simulink model "Tv_VSI"  (Simulink 8.1)
settings: Solver=ode23t  StartTime=0.0  StopTime=0.5  MaxStep=25e-6  RelTol=1e-4  AbsTol=1e-5
values from neighbouring files (symbols this model uses):
  C = 1*31.5e-6    (= 3.15e-05)    [TVSI_vil_tf_cal_sim_comp_frd_model.m]    (also in VSI_ol_init.m = 3.13e-05; VSI_ol_tf_cal_sim_comp_frd_model.m = 3.13e-05; Zac_VSI.m = 3.18e-05; Zdc_VSI.m)
  CR = .2    (= 0.2)    [TVSI_vil_tf_cal_sim_comp_frd_model.m]    (also in Zac_VSI.m = 1)
  Gdel = Gsvm    [TVSI_vil_tf_cal_sim_comp_frd_model.m]    (also in VSI_ol_init.m; VSI_ol_tf_cal_sim_comp_frd_model.m; Zac_VSI.m; Zdc_VSI.m)
  Ki = tf_filter_dq    [TVSI_vil_tf_cal_sim_comp_frd_model.m]    (also in VSI_ol_init.m; Zac_VSI.m; Zdc_VSI.m)
  kii = Kii_VSI/270    (= 0)    [TVSI_vil_tf_cal_sim_comp_frd_model.m]    (also in Zac_VSI.m; Zdc_VSI.m = 121.0095)
  kiv = Kiv_VSI    (= 523.598775598)    [TVSI_vil_tf_cal_sim_comp_frd_model.m]    (also in Zac_VSI.m = 78.5398163397; Zdc_VSI.m = 130.8997)
  kpi = Kpi_VSI/270    (= 0.0116355283466)    [TVSI_vil_tf_cal_sim_comp_frd_model.m]    (also in Zac_VSI.m = 0.00407243492132; Zdc_VSI.m = 0.0465)
  kpv = Kpv_VSI    (= 0.197920337176)    [TVSI_vil_tf_cal_sim_comp_frd_model.m]    (also in Zac_VSI.m = 0.0290283161192; Zdc_VSI.m = 0.0495)
  Kv = tf_filter_dq    [TVSI_vil_tf_cal_sim_comp_frd_model.m]    (also in VSI_ol_init.m; Zac_VSI.m; Zdc_VSI.m)
  L = 1.0e-3    (= 0.001)    [TVSI_vil_tf_cal_sim_comp_frd_model.m]    (also in VSI_ol_init.m; VSI_ol_tf_cal_sim_comp_frd_model.m; Zac_VSI.m = 0.000506643235509; Zdc_VSI.m)
  R = 12    [TVSI_vil_tf_cal_sim_comp_frd_model.m]    (also in VSI_ol_init.m = 15; VSI_ol_tf_cal_sim_comp_frd_model.m = 12000; Zac_VSI.m; Zdc_VSI.m)
  RL = 0.13    [TVSI_vil_tf_cal_sim_comp_frd_model.m]    (also in VSI_ol_init.m = 0.15; VSI_ol_tf_cal_sim_comp_frd_model.m = 0.15; Zac_VSI.m = 0.06; Zdc_VSI.m)
  Vdc = 270    [TVSI_vil_tf_cal_sim_comp_frd_model.m]    (also in VSI_ol_init.m; VSI_ol_tf_cal_sim_comp_frd_model.m; Zac_VSI.m; Zdc_VSI.m)
  Vdref = Vsdq(1)    [TVSI_vil_tf_cal_sim_comp_frd_model.m]    (also in VSI_ol_init.m; VSI_ol_tf_cal_sim_comp_frd_model.m; Zac_VSI.m; Zdc_VSI.m)
  Vqref = Vsdq(2)    [TVSI_vil_tf_cal_sim_comp_frd_model.m]    (also in VSI_ol_init.m; VSI_ol_tf_cal_sim_comp_frd_model.m; Zac_VSI.m; Zdc_VSI.m)
  w = 500*2*pi    (= 3141.59265359)    [JF_CMOD.m]    (also in JF_SMOD.m; TVSI_vil_tf_cal_sim_comp_frd_model.m = 376.991118431; VSI_ol_init.m = 2513.27412287; VSI_ol_tf_cal_sim_comp_frd_model.m = 376.991118431)
libraries: powerlib x28, cstblocks x12
settings Model: Creator=marko  LastModifiedBy=wenbo  BufferReuse=off
settings OptimizationCC: BlockReduction=off  InlineParams=on  BufferReuse=off
settings DebuggingCC: AlgebraicLoopMsg=none  SolverPrmCheckMsg=none  UnconnectedInputMsg=none  UnconnectedOutputMsg=none  UnconnectedLineMsg=none

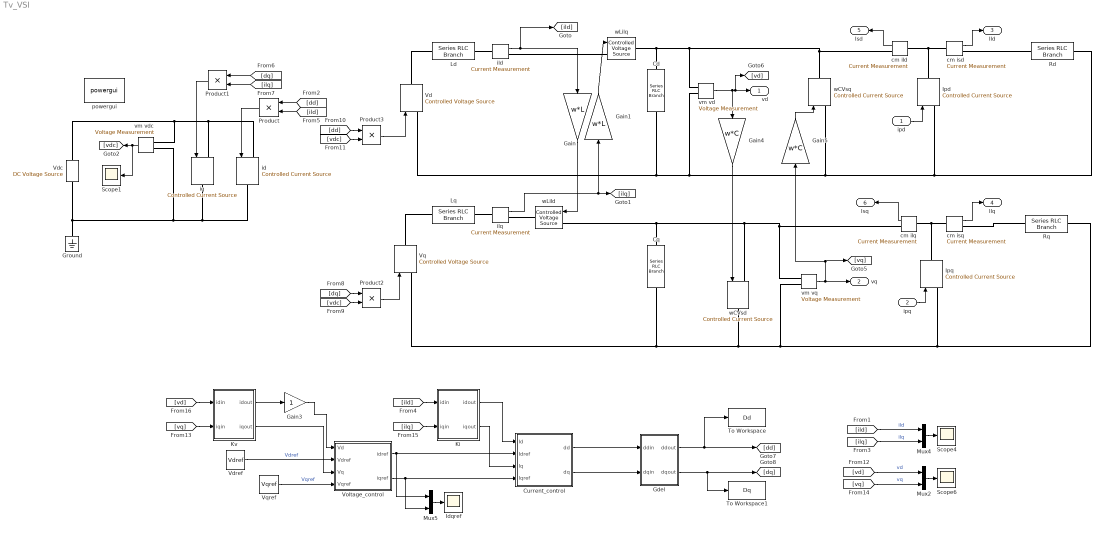
== system Tv_VSI ==
  ipd : Inport
  ipq : Inport  Port=2
  Cd : powerlib/Elements/Series RLC Branch  LConnTagsString=__new0  RConnTagsString=__new0  BranchType=RC  Resistance=CR  Inductance=1e-3  SetiL0=off  InitialCurrent=0  Capacitance=C  Setx0=off  InitialVoltage=0  Measurements=None
  Cq : powerlib/Elements/Series RLC Branch  LConnTagsString=__new0  RConnTagsString=__new0  BranchType=RC  Resistance=CR  Inductance=1e-3  SetiL0=off  InitialCurrent=0  Capacitance=C  Setx0=off  InitialVoltage=0  Measurements=None
  Current_control : Subsystem
  Gain : Gain  Gain=w*L
  Gain1 : Gain  Gain=w*L
  Gain3 : Gain
  Gain4 : Gain  Gain=w*C
  Gain5 : Gain  Gain=w*C
  Gdel : Subsystem
  Ground : powerlib/Elements/Ground  LConnTagsString=a
  Idqref : Scope
      settings: YMin=4.4  YMax=5.35  SaveName=ildq_matlab8
  Ipd : powerlib/Electrical Sources/Controlled Current Source  Initialize=on  Source_Type=AC  Amplitude=0  Phase=0  Frequency=0  Measurements=None
  Ipq : powerlib/Electrical Sources/Controlled Current Source  Initialize=on  Source_Type=AC  Amplitude=0  Phase=0  Frequency=0  Measurements=None
  Ki : Subsystem
  Kv : Subsystem
  Ld : powerlib/Elements/Series RLC Branch  LConnTagsString=__new0  RConnTagsString=__new0  BranchType=RL  Resistance=RL  Inductance=L  SetiL0=off  InitialCurrent=0  Capacitance=1e-6  Setx0=off  InitialVoltage=0  Measurements=None
  Lq : powerlib/Elements/Series RLC Branch  LConnTagsString=__new0  RConnTagsString=__new0  BranchType=RL  Resistance=RL  Inductance=L  SetiL0=off  InitialCurrent=0  Capacitance=1e-6  Setx0=off  InitialVoltage=0  Measurements=None
  Mux2 : Mux  Inputs=2
  Mux4 : Mux  Inputs=2
  Mux5 : Mux  Inputs=2
  Product{,1..3} (4 alike) : Product  RndMeth=Zero
  Rd : powerlib/Elements/Series RLC Branch  LConnTagsString=__new0  RConnTagsString=__new0  BranchType=R  Resistance=R  Inductance=1e-3  SetiL0=off  InitialCurrent=0  Capacitance=1e-6  Setx0=off  InitialVoltage=0  Measurements=None
  Rq : powerlib/Elements/Series RLC Branch  LConnTagsString=__new0  RConnTagsString=__new0  BranchType=R  Resistance=R  Inductance=1e-3  SetiL0=off  InitialCurrent=0  Capacitance=1e-6  Setx0=off  InitialVoltage=0  Measurements=None
  Scope1 : Scope
      settings: YMin=270  YMax=270  SaveName=ildq_matlab
  Scope4 : Scope
      settings: YMin=-0.25  YMax=5.25  SaveName=ildq_matlab3
  Scope6 : Scope
      settings: YMin=-10  YMax=130  SaveName=ildq_matlab4
  To Workspace : ToWorkspace  VariableName=Dd  SampleTime=-1
  To Workspace1 : ToWorkspace  VariableName=Dq  SampleTime=-1
  Vd : powerlib/Electrical Sources/Controlled Voltage Source  Initialize=on  Source_Type=DC  Amplitude=0  Phase=0  Frequency=0  Measurements=None
  Vdc : powerlib/Electrical Sources/DC Voltage Source  Amplitude=Vdc  Measurements=None
  Vdref : Constant  Value=Vdref
  Voltage_control : Subsystem
  Vq : powerlib/Electrical Sources/Controlled Voltage Source  Initialize=on  Source_Type=DC  Amplitude=0  Phase=0  Frequency=0  Measurements=None
  Vqref : Constant  Value=Vqref
  cm ild : powerlib/Measurements/Current Measurement  PhasorSimulation=off  OutputType=Complex  PSBequivalent=0
  cm ilq : powerlib/Measurements/Current Measurement  PhasorSimulation=off  OutputType=Complex  PSBequivalent=0
  cm isd : powerlib/Measurements/Current Measurement  PhasorSimulation=off  OutputType=Complex  PSBequivalent=0
  cm isq : powerlib/Measurements/Current Measurement  PhasorSimulation=off  OutputType=Complex  PSBequivalent=0
  id : powerlib/Electrical Sources/Controlled Current Source  Initialize=on  Source_Type=DC  Amplitude=0  Phase=0  Frequency=0  Measurements=None
  ild : powerlib/Measurements/Current Measurement  PhasorSimulation=off  OutputType=Complex  PSBequivalent=0
  ilq : powerlib/Measurements/Current Measurement  PhasorSimulation=off  OutputType=Complex  PSBequivalent=0
  iq : powerlib/Electrical Sources/Controlled Current Source  Initialize=on  Source_Type=DC  Amplitude=0  Phase=0  Frequency=0  Measurements=None
  powergui : powerlib/powergui  Priority=1  SimulationMode=Continuous  SolverType=Tustin  SampleTime=50e-6  frequency=60  SPID=off  DisableSnubberDevices=off  DisableRonSwitches=off  DisableVfSwitches=off  SwTol=0  Interpol=off  DisplayEquations=off  frequencyindice=0  Pbase=100e6  ErrMax=1e-4  Iterations=50  UnitsV=kV  UnitsW=MW  FunctionMessages=off  echomessages=off  HookPort=off  EnableUseOfTLC=off  x0status=blocks  RestoreLinks=warning  ResistiveCurrentMeasurement=off  Frange=[0:2:500]  Ylog=off  Xlog=on  ShowGrid=off  save=off  variable=ZData  ZoomFFT=on  StartTime=0.0  cycles=1  DisplayStyle=1  fundamental=60  FreqAxis=off  MaxFrequency=1000  frequencyindicesteady=1  RmsSteady=1  display=off  Ts=0  methode=off
  vm vd : powerlib/Measurements/Voltage Measurement  PhasorSimulation=off  OutputType=Complex  PSBequivalent=0
  vm vdc : powerlib/Measurements/Voltage Measurement  PhasorSimulation=off  OutputType=Complex  PSBequivalent=0
  vm vq : powerlib/Measurements/Voltage Measurement  PhasorSimulation=off  OutputType=Complex  PSBequivalent=0
  wCVsd : powerlib/Electrical Sources/Controlled Current Source  Initialize=on  Source_Type=DC  Amplitude=0  Phase=0  Frequency=0  Measurements=None
  wCVsq : powerlib/Electrical Sources/Controlled Current Source  Initialize=on  Source_Type=DC  Amplitude=0  Phase=0  Frequency=0  Measurements=None
  wLild : powerlib/Electrical Sources/Controlled Voltage Source  Initialize=on  Source_Type=DC  Amplitude=0  Phase=0  Frequency=0  Measurements=None
  wLilq : powerlib/Electrical Sources/Controlled Voltage Source  Initialize=on  Source_Type=DC  Amplitude=0  Phase=0  Frequency=0  Measurements=None
  vd : Outport
  vq : Outport  Port=2
  Ild : Outport  Port=3
  Ilq : Outport  Port=4
  Isd : Outport  Port=5
  Isq : Outport  Port=6
  wires:
  [ild] -> Mux4/1  "ild"
  [ilq] -> Mux4/2  "ilq"
  Mux4/1 -> Scope4/1
  [vd] -> Mux2/1  "vd"
  [vq] -> Mux2/2  "vq"
  Mux2/1 -> Scope6/1
  Voltage_control/2(iqref) -> Mux5/2, Current_control/4(Iqref)
  Gdel/1(ddout) -> [dd], To Workspace/1
  Gdel/2(dqout) -> [dq], To Workspace1/1
  Vqref/1 -> Voltage_control/4(Vqref)  "Vqref"
  Vdref/1 -> Voltage_control/2(Vdref)  "Vdref"
  Voltage_control/1(idref) -> Mux5/1, Current_control/2(Idref)
  Mux5/1 -> Idqref/1
  [ild] -> Ki/1(idin)
  [ilq] -> Ki/2(iqin)
  Ki/1(idout) -> Current_control/1(Id)
  Ki/2(iqout) -> Current_control/3(Iq)
  Current_control/1(dd) -> Gdel/1(ddin)
  Current_control/2(dq) -> Gdel/2(dqin)
  [vd] -> Kv/1(idin)
  [vq] -> Kv/2(iqin)
  Kv/2(iqout) -> Voltage_control/3(Vq)
  Kv/1(idout) -> Gain3/1
  Gain3/1 -> Voltage_control/1(Vd)
  Product1/1 -> iq/1
  [dq] -> Product2/1
  [vdc] -> Product2/2
  Product2/1 -> Vq/1
  [dd] -> Product3/1
  [vdc] -> Product3/2
  Product3/1 -> Vd/1
  vm vd/1 -> vd/1, [vd], Gain4/1
  vm vq/1 -> vq/1, Gain5/1, [vq]
  vm vdc/1 -> [vdc], Scope1/1
  ilq/1 -> [ilq], Gain1/1
  ild/1 -> Gain/1, [ild]
  Gain5/1 -> wCVsq/1
  [dd] -> Product/1
  [ild] -> Product/2
  [dq] -> Product1/1
  [ilq] -> Product1/2
  Product/1 -> id/1
  Gain/1 -> wLild/1
  Gain1/1 -> wLilq/1
  Gain4/1 -> wCVsd/1
  ipd/1 -> Ipd/1
  cm ild/1 -> Isd/1
  cm isd/1 -> Ild/1
  ipq/1 -> Ipq/1
  cm ilq/1 -> Isq/1
  cm isq/1 -> Ilq/1
  connections:
  vm vq/LConn2 -- Rq/RConn1 -- Ipq/LConn1 -- wCVsd/RConn1 -- Vq/LConn1 -- Cq/RConn1
  vm vdc/LConn2 -- Ground/LConn1 -- Vdc/LConn1 -- iq/RConn1 -- id/RConn1
  vm vq/LConn1 -- cm ilq/RConn1 -- wCVsd/LConn1 -- wLild/LConn1 -- Cq/LConn1
  vm vdc/LConn1 -- Vdc/RConn1 -- id/LConn1 -- iq/LConn1
  vm vd/LConn1 -- cm ild/RConn1 -- wCVsq/RConn1 -- Cd/LConn1 -- wLilq/RConn1
  vm vd/LConn2 -- Ipd/LConn1 -- Rd/RConn1 -- wCVsq/LConn1 -- Vd/LConn1 -- Cd/RConn1
  cm ild/LConn1 -- Ipd/RConn1 -- cm isd/LConn1
  cm ilq/LConn1 -- Ipq/RConn1 -- cm isq/LConn1
  wLild/RConn1 -- ilq/RConn1
  Ld/LConn1 -- Vd/RConn1
  ilq/LConn1 -- Lq/LConn1
  cm isd/RConn1 -- Rd/LConn1
  Lq/RConn1 -- Vq/RConn1
  wLilq/LConn1 -- ild/RConn1
  cm isq/RConn1 -- Rq/LConn1
  ild/LConn1 -- Ld/RConn1

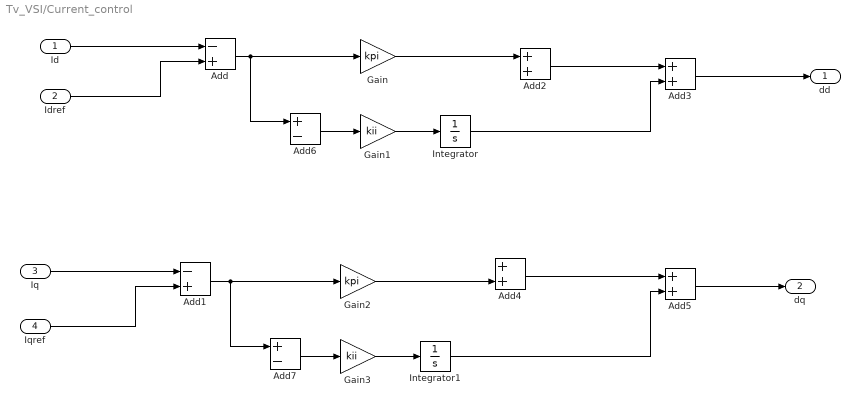
== system Tv_VSI/Current_control ==
  Id : Inport
  Idref : Inport  Port=2
  Iq : Inport  Port=3
  Iqref : Inport  Port=4
  Add : Sum  Inputs=-+
  Add1 : Sum  Inputs=-+
  Add{2..5} (4 alike) : Sum
  Add6 : Sum  Inputs=+-
  Add7 : Sum  Inputs=+-
  Gain : Gain  Gain=kpi
  Gain1 : Gain  Gain=kii
  Gain2 : Gain  Gain=kpi
  Gain3 : Gain  Gain=kii
  Integrator : Integrator
  Integrator1 : Integrator
  dd : Outport
  dq : Outport  Port=2
  wires:
  Id/1 -> Add/1
  Idref/1 -> Add/2
  Iq/1 -> Add1/1
  Iqref/1 -> Add1/2
  Add/1 -> Gain/1, Add6/1
  Gain1/1 -> Integrator/1
  Integrator/1 -> Add3/2
  Gain/1 -> Add2/1
  Add1/1 -> Gain2/1, Add7/1
  Gain3/1 -> Integrator1/1
  Gain2/1 -> Add4/2
  Add4/1 -> Add5/1
  Integrator1/1 -> Add5/2
  Add3/1 -> dd/1
  Add6/1 -> Gain1/1
  Add7/1 -> Gain3/1
  Add5/1 -> dq/1
  Add2/1 -> Add3/1

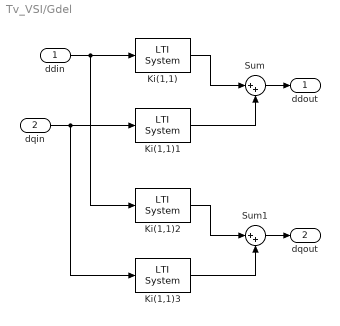
== system Tv_VSI/Gdel ==
  ddin : Inport
  dqin : Inport  Port=2
  Ki(1,1) : cstblocks/LTI System  sys=Gdel(1,1)  IC=[]
  Ki(1,1)1 : cstblocks/LTI System  sys=Gdel(1,2)  IC=[]
  Ki(1,1)2 : cstblocks/LTI System  sys=Gdel(2,1)  IC=[]
  Ki(1,1)3 : cstblocks/LTI System  sys=Gdel(2,2)  IC=[]
  Sum : Sum  Inputs=|++
  Sum1 : Sum  Inputs=|++
  ddout : Outport
  dqout : Outport  Port=2
  wires:
  Ki(1,1)/1 -> Sum/1
  Ki(1,1)1/1 -> Sum/2
  Ki(1,1)2/1 -> Sum1/1
  Ki(1,1)3/1 -> Sum1/2
  ddin/1 -> Ki(1,1)/1, Ki(1,1)2/1
  dqin/1 -> Ki(1,1)1/1, Ki(1,1)3/1
  Sum/1 -> ddout/1
  Sum1/1 -> dqout/1

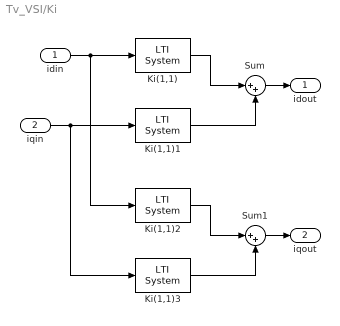
== system Tv_VSI/Ki ==
  idin : Inport
  iqin : Inport  Port=2
  Ki(1,1) : cstblocks/LTI System  sys=Ki(1,1)  IC=[]
  Ki(1,1)1 : cstblocks/LTI System  sys=Ki(1,2)  IC=[]
  Ki(1,1)2 : cstblocks/LTI System  sys=Ki(2,1)  IC=[]
  Ki(1,1)3 : cstblocks/LTI System  sys=Ki(2,2)  IC=[]
  Sum : Sum  Inputs=|++
  Sum1 : Sum  Inputs=|++
  idout : Outport
  iqout : Outport  Port=2
  wires:
  Ki(1,1)/1 -> Sum/1
  Ki(1,1)1/1 -> Sum/2
  Ki(1,1)2/1 -> Sum1/1
  Ki(1,1)3/1 -> Sum1/2
  idin/1 -> Ki(1,1)/1, Ki(1,1)2/1
  iqin/1 -> Ki(1,1)1/1, Ki(1,1)3/1
  Sum/1 -> idout/1
  Sum1/1 -> iqout/1

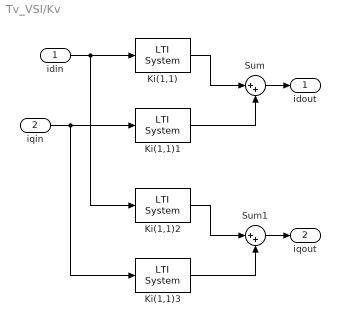
== system Tv_VSI/Kv ==
  idin : Inport
  iqin : Inport  Port=2
  Ki(1,1) : cstblocks/LTI System  sys=Kv(1,1)  IC=[]
  Ki(1,1)1 : cstblocks/LTI System  sys=Kv(1,2)  IC=[]
  Ki(1,1)2 : cstblocks/LTI System  sys=Kv(2,1)  IC=[]
  Ki(1,1)3 : cstblocks/LTI System  sys=Kv(2,2)  IC=[]
  Sum : Sum  Inputs=|++
  Sum1 : Sum  Inputs=|++
  idout : Outport
  iqout : Outport  Port=2
  wires:
  Sum1/1 -> iqout/1
  Sum/1 -> idout/1
  iqin/1 -> Ki(1,1)3/1, Ki(1,1)1/1
  idin/1 -> Ki(1,1)2/1, Ki(1,1)/1
  Ki(1,1)3/1 -> Sum1/2
  Ki(1,1)2/1 -> Sum1/1
  Ki(1,1)1/1 -> Sum/2
  Ki(1,1)/1 -> Sum/1

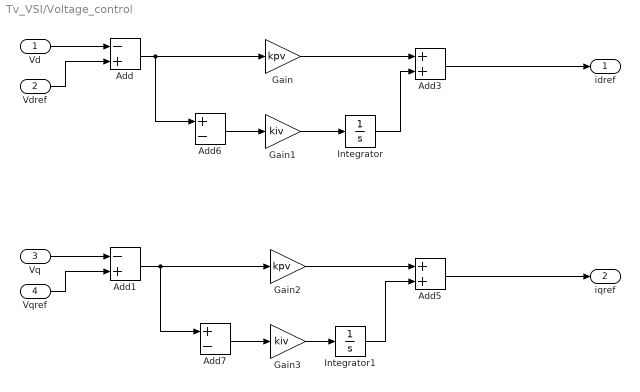
== system Tv_VSI/Voltage_control ==
  Vd : Inport
  Vdref : Inport  Port=2
  Vq : Inport  Port=3
  Vqref : Inport  Port=4
  Add : Sum  Inputs=-+
  Add1 : Sum  Inputs=-+
  Add3 : Sum
  Add5 : Sum
  Add6 : Sum  Inputs=+-
  Add7 : Sum  Inputs=+-
  Gain : Gain  Gain=kpv
  Gain1 : Gain  Gain=kiv
  Gain2 : Gain  Gain=kpv
  Gain3 : Gain  Gain=kiv
  Integrator : Integrator
  Integrator1 : Integrator
  idref : Outport
  iqref : Outport  Port=2
  wires:
  Add3/1 -> idref/1
  Add7/1 -> Gain3/1
  Add6/1 -> Gain1/1
  Add5/1 -> iqref/1
  Integrator1/1 -> Add5/2
  Gain2/1 -> Add5/1
  Gain3/1 -> Integrator1/1
  Add1/1 -> Add7/1, Gain2/1
  Gain/1 -> Add3/1
  Integrator/1 -> Add3/2
  Gain1/1 -> Integrator/1
  Add/1 -> Add6/1, Gain/1
  Vqref/1 -> Add1/2
  Vq/1 -> Add1/1
  Vdref/1 -> Add/2
  Vd/1 -> Add/1
